simulink model "MEMS_model"  (R2013a)
settings: Solver=ode3  StartTime=0.0  StopTime=20.0  FixedStep=1/50  RelTol=1e-3
values from neighbouring files (symbols this model uses):
  gyro_bias = mean(real_gyro_data) * v2dps    [mems_model_test.m]
  lower_saturation = -2^15    (= -32768)    [mems_model_test.m]
  rate_noise_density = AVAR(samp_freq)    [mems_model_test.m]
  samp_freq = 50    [mems_model_test.m]
  sensitivity = 0.010    (= 0.01)    [mems_model_test.m]
  upper_saturation = 2^15    (= 32768)    [mems_model_test.m]
  w = 12.5*2*pi    (= 78.5398163397)    [mems_model_test.m]
  wn = 1000*2*pi    (= 6283.18530718)    [mems_model_test.m]
  z = zeta    [mems_model_test.m]
  zeta = sqrt(2)/2    [mems_model_test.m]
libraries: simulink x1
settings Model: Creator=Alberto  LastModifiedBy=Alberto

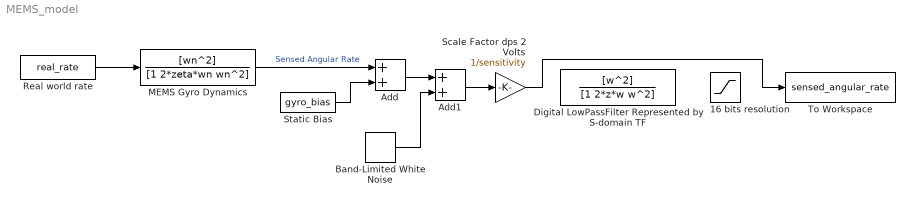
== system MEMS_model ==
  16 bits resolution : Saturate  UpperLimit=upper_saturation  LowerLimit=lower_saturation
  Add : Sum
  Add1 : Sum
  Band-Limited White Noise : simulink/Sources/Band-Limited White Noise  Cov=[rate_noise_density^2]  Ts=1/samp_freq  seed=[1]
  Digital LowPassFilter Represented by S-domain TF : TransferFcn  Numerator=[w^2]  Denominator=[1 2*z*w w^2]
  MEMS Gyro Dynamics : TransferFcn  Numerator=[wn^2]  Denominator=[1 2*zeta*wn wn^2]
  Real world rate : FromWorkspace  VariableName=real_rate  SampleTime=0
  Scale Factor dps 2 Volts : Gain  Gain=1/sensitivity
  Static Bias : Constant  Value=gyro_bias
  To Workspace : ToWorkspace  VariableName=sensed_angular_rate  SampleTime=-1
  wires:
  Real world rate/1 -> MEMS Gyro Dynamics/1
  Scale Factor dps 2 Volts/1 -> To Workspace/1
  MEMS Gyro Dynamics/1 -> Add/1  "Sensed Angular Rate"
  Add/1 -> Add1/1
  Static Bias/1 -> Add/2
  Add1/1 -> Scale Factor dps 2 Volts/1
  Band-Limited White Noise/1 -> Add1/2
